simulink model "testDataLogger"  (R2014a)
settings: Solver=FixedStepDiscrete  StartTime=0.0  StopTime=Inf  FixedStep=0.001  RelTol=1e-3
PreLoadFcn:
  | testDataLoggerLocal_Initialize();
InitFcn:
  | testDataLoggerLocal_Initialize();
undefined symbols (not defined in the file or in its folder): macaddr
libraries: simulink x4, libButtons x3, libBusSerialize x3, xpcnetworkbufferlib x1, xpcethernetlib x1
settings Model: xpc_rtwmakecfg_data=_xpcnblib__xpcetherlib__xpcether8255xlib__xpcetherGbElib_  SimulationMode=external  BufferReuse=off  Creator=shenoylab  LastModifiedBy=shenoylab
settings SolverCC: EnableConcurrentExecution=on
settings DataIOCC: SignalLoggingSaveFormat=ModelDataLogs
settings OptimizationCC: BlockReduction=off  OptimizeBlockIOStorage=off  BufferReuse=off  GlobalBufferReuse=off  ExpressionFolding=off  LocalBlockOutputs=off
settings DebuggingCC: SaveWithDisabledLinksMsg=none  MultiTaskDSMMsg=warning  MultiTaskCondExecSysMsg=none  StateNameClashWarn=warning
settings HardwareCC: ProdIntDivRoundTo=Zero  ProdEndianess=LittleEndian  ProdHWDeviceType=Generic->32-bit x86 compatible
settings RTWCC: SystemTargetFile=slrt.tlc  TemplateMakefile=slrt_default_tmf  Description=Simulink Real-Time  GenerateReport=on  ProcessScript=slrt_make_rtw_hook  LaunchReport=on  IncludeERTFirstTime=on  RTWCompilerOptimization=On
settings CodeAppCC: MATLABSourceComments=on
settings SimulinkRealTimeCC: GeneratePreprocessorConditionals=Disable all  EnableShiftOperators=on

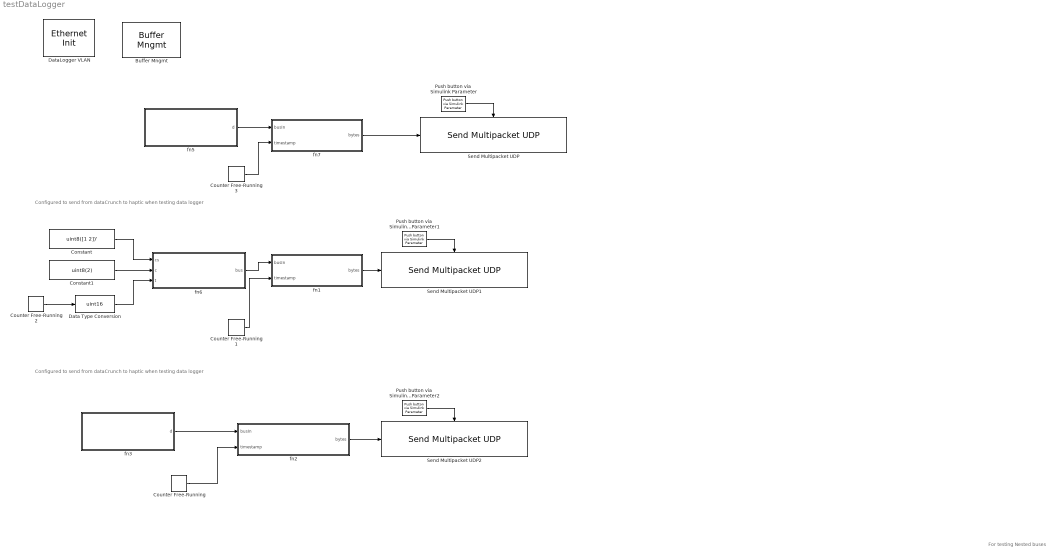
== system testDataLogger ==
  note: Configured to send from dataCrunch to haptic when testing data logger
  note: For testing Nested buses
  note: Configured to send from dataCrunch to haptic when testing data logger
  "Buffer Mngmt " : xpcnetworkbufferlib/Buffer Mngmt   Priority=-1  SampleTime=-1  PoolSizes=[256 512 1024 2048]  ShowTune=off
  Constant : Constant  Value=uint8([1 2])'
  Constant1 : Constant  Value=uint8(2)
  Counter Free-Running : simulink/Sources/Counter Free-Running  NumBits=32  tsamp=-1
  Counter Free-Running1 : simulink/Sources/Counter Free-Running  NumBits=32  tsamp=-1
  Counter Free-Running2 : simulink/Sources/Counter Free-Running  NumBits=16  tsamp=-1
  Counter Free-Running3 : simulink/Sources/Counter Free-Running  NumBits=32  tsamp=-1
  Data Type Conversion : DataTypeConversion  OutDataTypeStr=uint16
  DataLogger VLAN : xpcethernetlib/Ethernet Init   Priority=-1  ID=2  Driver=Intel 8255x  Bus=3  Slot=5  SampleTime=-1  AddressSource=EEPROM  MAC=macaddr('00:00:00:00:00:00')  TxSA=off  RxPromiscuous=off  Multicast={}  RxBad=off  RxShort=off  MaxMTU=1518  TxThreshold=224  TxBuffers=256  RxBuffers=64  ShowTune=off  NumRxBlks=1
  Push button via Simulink Parameter : libButtons/Push button via Simulink Parameter  paramName=param1  Ts=0.001
  Push button via Simulink Parameter1 : libButtons/Push button via Simulink Parameter  paramName=param2  Ts=0.001
  Push button via Simulink Parameter2 : libButtons/Push button via Simulink Parameter  paramName=param3  Ts=0.001
  Send Multipacket UDP : libBusSerialize/Send Multipacket UDP  transmitId=2  sourceIP=[192 168 1 1]  sourcePort=20000  destIP=[192 168 1 255]  destPort=25000  destMac=macaddr('ff:ff:ff:ff:ff:ff')  ID=2  prependHeader=on
  Send Multipacket UDP1 : libBusSerialize/Send Multipacket UDP  transmitId=2  sourceIP=[192 168 1 1]  sourcePort=20000  destIP=[192 168 1 255]  destPort=25000  destMac=macaddr('ff:ff:ff:ff:ff:ff')  ID=2  prependHeader=on
  Send Multipacket UDP2 : libBusSerialize/Send Multipacket UDP  transmitId=3  sourceIP=[192 168 1 1]  sourcePort=20000  destIP=[192 168 1 255]  destPort=25000  destMac=macaddr('ff:ff:ff:ff:ff:ff')  ID=2  prependHeader=on
  fn1 : MATLAB Function  AncestorBlock=libBusSerialize/fn2  TreatAsAtomicUnit=on  mask(BusSerialize: serialize block){busType=Bus: TestBusOuter, groupType=Parameters, groupName='testBusOuter'}
      mask prompts: busType "Bus Type"; groupType "Group Type"; groupName "Group Name"
      mask help: Select the bus type below to serialize.
      mask init:
      | BusSerialize.maskSerializeWithDataLoggerHeaderBlockUpdate(gcb)
  fn2 : MATLAB Function  AncestorBlock=libBusSerialize/fn2  TreatAsAtomicUnit=on  mask(BusSerialize: serialize block){busType=Bus: DataLoggerControlBus, groupType=Control, groupName='control'}
      mask prompts: busType "Bus Type"; groupType "Group Type"; groupName "Group Name"
      mask help: Select the bus type below to serialize.
      mask init:
      | BusSerialize.maskSerializeWithDataLoggerHeaderBlockUpdate(gcb)
  fn3 : MATLAB Function  TreatAsAtomicUnit=on
  fn5 : MATLAB Function  TreatAsAtomicUnit=on
  fn6 : MATLAB Function  TreatAsAtomicUnit=on
  fn7 : MATLAB Function  AncestorBlock=libBusSerialize/fn2  TreatAsAtomicUnit=on  mask(BusSerialize: serialize block){busType=Bus: TestBus, groupType=Analog Channels, groupName='analog'}
      mask prompts: busType "Bus Type"; groupType "Group Type"; groupName "Group Name"
      mask help: Select the bus type below to serialize.
      mask init:
      | BusSerialize.maskSerializeWithDataLoggerHeaderBlockUpdate(gcb)
  wires:
  fn6/1(bus) -> fn1/1(busIn)
  Constant/1 -> fn6/1(cs)
  Constant1/1 -> fn6/2(c)
  Data Type Conversion/1 -> fn6/3(t)
  Counter Free-Running2/1 -> Data Type Conversion/1
  fn1/1(bytes) -> Send Multipacket UDP1/1
  fn3/1(d) -> fn2/1(busIn)
  fn2/1(bytes) -> Send Multipacket UDP2/1
  Counter Free-Running/1 -> fn2/2(timestamp)
  Counter Free-Running1/1 -> fn1/2(timestamp)
  fn5/1(d) -> fn7/1(busIn)
  Counter Free-Running3/1 -> fn7/2(timestamp)
  Push button via Simulink Parameter/1 -> Send Multipacket UDP/Enable
  fn7/1(bytes) -> Send Multipacket UDP/1
  Push button via Simulink Parameter1/1 -> Send Multipacket UDP1/Enable
  Push button via Simulink Parameter2/1 -> Send Multipacket UDP2/Enable

== matlab function testDataLogger/fn1 ==
  data: busIn input Bus: TestBusOuter size=1; bytes output uint8 size=154; timestamp input uint32 size=1
function bytes = dataLoggerSerialize(busIn, timestamp)
%#codegen
    bytes = testDataLoggerLib.serializeBusWithDataLoggerHeader_TestBusOuter(busIn, uint8(2), uint8('testBusOuter'), timestamp);
end

== matlab function testDataLogger/fn2 ==
  data: busIn input Bus: DataLoggerControlBus size=1; bytes output uint8 size=253; timestamp input uint32 size=1
function bytes = dataLoggerSerialize(busIn, timestamp)
%#codegen
    bytes = testDataLoggerLib.serializeBusWithDataLoggerHeader_DataLoggerControlBus(busIn, uint8(1), uint8('control'), timestamp);
end

== matlab function testDataLogger/fn3 ==
  data: d output Bus: DataLoggerControlBus size=1
function d = createBus()

d.dataStore = uint8('testStore')';
d.subject = uint8('testSubj')';
d.protocol =  uint8('testProto')';
d.protocolVersion = uint32(20140428);
d.saveTag = uint32(1);
d.nextTrial = uint8(1);

== matlab function testDataLogger/fn6 ==
  data: bus output Bus: TestBusOuter size=1; cs input uint8; c input uint8; t input uint16
function bus = createBus(cs, c, t)

P1.centerSize = uint8(cs);
P1.holdWindowCenter = uint8(c);
P1.holdWindowTarget = uint16(t);

bus.val1 = uint8(3);
bus.val2 = uint8('hello')';
bus.nested = P1;

== matlab function testDataLogger/fn5 ==
  data: d output Bus: TestBus size=1
function d = createBus()

d.centerSize = ones(255, 20, 'uint8');
d.holdWindowCenter = uint8(15);
d.holdWindowTarget = uint8('helloWorld')';

== matlab function testDataLogger/fn7 ==
  data: busIn input Bus: TestBus size=1; bytes output uint8 size=5236; timestamp input uint32 size=1
function bytes = dataLoggerSerialize(busIn, timestamp)
%#codegen
    bytes = testDataLoggerLib.serializeBusWithDataLoggerHeader_TestBus(busIn, uint8(3), uint8('analog'), timestamp);
end
